simulink model "MBNLC_cascade_rov"  (Simulink 6.0)
settings: Solver=ode45  StartTime=0.0  StopTime=650  RelTol=1e-3
undefined symbols (not defined in the file): B, DQ, DQL, I, m, M, Ma, MaL, MaU, rg, sigbuilder_block, T, W, xb, xg, Xudot, yb, yg, Yvdot, zb, zg, Zwdot
libraries: simulink_extras x12, simulink x8
(part 3 of 3)

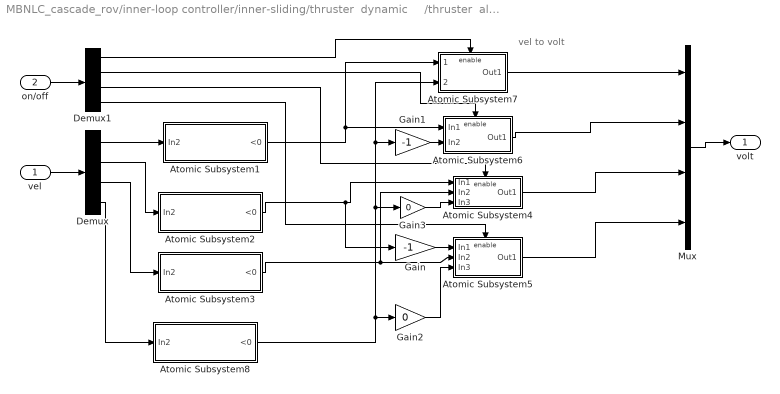
== system MBNLC_cascade_rov/inner-loop controller/inner-sliding/thruster  dynamic     /thruster  alloc. /thruster  allocation control1/thruster allocation  ==
  note: vel to volt
  vel : Inport  Port=1  LatchInput=off
  on/off : Inport  Port=2  LatchInput=off
  Atomic Subsystem1 : Subsystem  TreatAsAtomicUnit=on
      mask Display: disp('check x >0, send \n signal to thrusters ')
  Atomic Subsystem2 : Subsystem  TreatAsAtomicUnit=on
      mask Display: disp('check y >0, send \n signal to thrusters ')
  Atomic Subsystem3 : Subsystem  TreatAsAtomicUnit=on
      mask Display: disp('check z >0, send \n signal to thrusters ')
  Atomic Subsystem4 : Subsystem  TreatAsAtomicUnit=on
      mask Display: disp('activate T3')
  Atomic Subsystem5 : Subsystem  TreatAsAtomicUnit=on
      mask Display: disp('activate T4')
  Atomic Subsystem6 : Subsystem  TreatAsAtomicUnit=on
      mask Display: disp('activate T2')
  Atomic Subsystem7 : Subsystem  TreatAsAtomicUnit=on
      mask Display: disp('activate T1')
  Atomic Subsystem8 : Subsystem  TreatAsAtomicUnit=on
      mask Display: disp('check yaw >0, send \n signal to thrusters ')
  Demux : Demux
  Demux1 : Demux
  Gain : Gain  Gain=-1
  Gain1 : Gain  Gain=-1
  Gain2 : Gain  Gain=0
  Gain3 : Gain  Gain=0
  Mux : Mux
  volt : Outport
  wires:
  Demux/1 -> Atomic Subsystem1/1(In2)
  Demux/2 -> Atomic Subsystem2/1(In2)
  Demux/3 -> Atomic Subsystem3/1(In2)
  Atomic Subsystem7/1(Out1) -> Mux/1
  vel/1 -> Demux/1
  Demux/4 -> Atomic Subsystem8/1(In2)
  on/off/1 -> Demux1/1
  Mux/1 -> volt/1
  Atomic Subsystem6/1(Out1) -> Mux/2
  Atomic Subsystem4/1(Out1) -> Mux/3
  Atomic Subsystem5/1(Out1) -> Mux/4
  Atomic Subsystem1/1(<0) -> Atomic Subsystem7/1(1), Atomic Subsystem6/1(In1)
  Atomic Subsystem2/1(<0) -> Atomic Subsystem4/1(In1), Gain/1
  Atomic Subsystem3/1(<0) -> Atomic Subsystem4/2(In2), Atomic Subsystem5/2(In2)
  Gain/1 -> Atomic Subsystem5/1(In1)
  Atomic Subsystem8/1(<0) -> Atomic Subsystem7/2(2), Gain1/1, Gain3/1, Gain2/1
  Gain1/1 -> Atomic Subsystem6/2(In2)
  Gain2/1 -> Atomic Subsystem5/3(In3)
  Demux1/1 -> Atomic Subsystem7/Enable
  Demux1/2 -> Atomic Subsystem6/Enable
  Demux1/3 -> Atomic Subsystem4/Enable
  Demux1/4 -> Atomic Subsystem5/Enable
  Gain3/1 -> Atomic Subsystem4/3(In3)

== system MBNLC_cascade_rov/inner-loop controller/inner -PI-decouple /thruster  dynamic     /thruster  alloc. /thruster  allocation control1/thruster allocation /Atomic Subsystem1 ==
  In2 : Inport  Port=1  LatchInput=off
  Abs : Abs
  Product1 : Product  OutDataTypeMode=double  SaturateOnIntegerOverflow=on  RndMeth=Zero
  Product5 : Product  OutDataTypeMode=double  SaturateOnIntegerOverflow=on  RndMeth=Zero
  Sign1 : Signum
  Switch1 : Switch  Threshold=1  SaturateOnIntegerOverflow=on  InputSameDT=on
  <0 : Outport
  wires:
  Sign1/1 -> Product1/2, Product5/1, Switch1/2
  Product1/1 -> Switch1/1
  Product5/1 -> Switch1/3
  Switch1/1 -> <0/1
  In2/1 -> Sign1/1, Product1/1, Abs/1
  Abs/1 -> Product5/2

== system MBNLC_cascade_rov/inner-loop controller/inner -PI-decouple /thruster  dynamic     /thruster  alloc. /thruster  allocation control1/thruster allocation /Atomic Subsystem2 ==
  In2 : Inport  Port=1  LatchInput=off
  Abs : Abs
  Product1 : Product  OutDataTypeMode=double  SaturateOnIntegerOverflow=on  RndMeth=Zero
  Product5 : Product  OutDataTypeMode=double  SaturateOnIntegerOverflow=on  RndMeth=Zero
  Sign1 : Signum
  Switch1 : Switch  Threshold=1  SaturateOnIntegerOverflow=on  InputSameDT=on
  <0 : Outport
  wires:
  In2/1 -> Sign1/1, Product1/1, Abs/1
  Sign1/1 -> Switch1/2, Product1/2, Product5/1
  Product1/1 -> Switch1/1
  Product5/1 -> Switch1/3
  Switch1/1 -> <0/1
  Abs/1 -> Product5/2

== system MBNLC_cascade_rov/inner-loop controller/inner -PI-decouple /thruster  dynamic     /thruster  alloc. /thruster  allocation control1/thruster allocation /Atomic Subsystem3 ==
  In2 : Inport  Port=1  LatchInput=off
  Abs : Abs
  Product1 : Product  OutDataTypeMode=double  SaturateOnIntegerOverflow=on  RndMeth=Zero
  Product5 : Product  OutDataTypeMode=double  SaturateOnIntegerOverflow=on  RndMeth=Zero
  Sign1 : Signum
  Switch1 : Switch  Threshold=1  SaturateOnIntegerOverflow=on  InputSameDT=on
  <0 : Outport
  wires:
  Sign1/1 -> Switch1/2, Product1/2, Product5/1
  Product1/1 -> Switch1/1
  Product5/1 -> Switch1/3
  Switch1/1 -> <0/1
  In2/1 -> Sign1/1, Product1/1, Abs/1
  Abs/1 -> Product5/2

== system MBNLC_cascade_rov/inner-loop controller/inner -PI-decouple /thruster  dynamic     /thruster  alloc. /thruster  allocation control1/thruster allocation /Atomic Subsystem4 ==
  In1 : Inport  Port=1  LatchInput=off
  In2 : Inport  Port=2  LatchInput=off
  In3 : Inport  Port=3  LatchInput=off
  Enable : EnablePort
  Subtract : Sum  Inputs=+++  OutScaling=2^-10
  Out1 : Outport
  wires:
  In1/1 -> Subtract/1
  In2/1 -> Subtract/2
  In3/1 -> Subtract/3
  Subtract/1 -> Out1/1

== system MBNLC_cascade_rov/inner-loop controller/inner -PI-decouple /thruster  dynamic     /thruster  alloc. /thruster  allocation control1/thruster allocation /Atomic Subsystem5 ==
  In1 : Inport  Port=1  LatchInput=off
  In2 : Inport  Port=2  LatchInput=off
  In3 : Inport  Port=3  LatchInput=off
  Enable : EnablePort
  Subtract : Sum  Inputs=+++  OutScaling=2^-10
  Out1 : Outport
  wires:
  In1/1 -> Subtract/1
  In2/1 -> Subtract/2
  In3/1 -> Subtract/3
  Subtract/1 -> Out1/1

== system MBNLC_cascade_rov/inner-loop controller/inner -PI-decouple /thruster  dynamic     /thruster  alloc. /thruster  allocation control1/thruster allocation /Atomic Subsystem6 ==
  In1 : Inport  Port=1  LatchInput=off
  In2 : Inport  Port=2  LatchInput=off
  Enable : EnablePort
  Subtract : Sum  OutScaling=2^-10
  Out1 : Outport
  wires:
  In1/1 -> Subtract/1
  In2/1 -> Subtract/2
  Subtract/1 -> Out1/1

== system MBNLC_cascade_rov/inner-loop controller/inner -PI-decouple /thruster  dynamic     /thruster  alloc. /thruster  allocation control1/thruster allocation /Atomic Subsystem7 ==
  1 : Inport  Port=1  LatchInput=off
  2 : Inport  Port=2  LatchInput=off
  Enable : EnablePort
  Subtract : Sum  OutScaling=2^-10
  Out1 : Outport
  wires:
  1/1 -> Subtract/1
  2/1 -> Subtract/2
  Subtract/1 -> Out1/1

== system MBNLC_cascade_rov/inner-loop controller/inner -PI-decouple /thruster  dynamic     /thruster  alloc. /thruster  allocation control1/thruster allocation /Atomic Subsystem8 ==
  In2 : Inport  Port=1  LatchInput=off
  Abs : Abs
  Product1 : Product  OutDataTypeMode=double  SaturateOnIntegerOverflow=on  RndMeth=Zero
  Product5 : Product  OutDataTypeMode=double  SaturateOnIntegerOverflow=on  RndMeth=Zero
  Sign1 : Signum
  Switch1 : Switch  Threshold=1  SaturateOnIntegerOverflow=on  InputSameDT=on
  <0 : Outport
  wires:
  In2/1 -> Sign1/1, Product1/1, Abs/1
  Sign1/1 -> Switch1/2, Product1/2, Product5/1
  Product1/1 -> Switch1/1
  Product5/1 -> Switch1/3
  Switch1/1 -> <0/1
  Abs/1 -> Product5/2

== system MBNLC_cascade_rov/inner-loop controller/inner -backstepping/thruster  dynamic     /thruster  alloc. /thruster  allocation control1/thruster allocation /Atomic Subsystem1 ==
  In2 : Inport  Port=1  LatchInput=off
  Abs : Abs
  Product1 : Product  OutDataTypeMode=double  SaturateOnIntegerOverflow=on  RndMeth=Zero
  Product5 : Product  OutDataTypeMode=double  SaturateOnIntegerOverflow=on  RndMeth=Zero
  Sign1 : Signum
  Switch1 : Switch  Threshold=1  SaturateOnIntegerOverflow=on  InputSameDT=on
  <0 : Outport
  wires:
  Sign1/1 -> Product1/2, Product5/1, Switch1/2
  Product1/1 -> Switch1/1
  Product5/1 -> Switch1/3
  Switch1/1 -> <0/1
  In2/1 -> Sign1/1, Product1/1, Abs/1
  Abs/1 -> Product5/2

== system MBNLC_cascade_rov/inner-loop controller/inner -backstepping/thruster  dynamic     /thruster  alloc. /thruster  allocation control1/thruster allocation /Atomic Subsystem2 ==
  In2 : Inport  Port=1  LatchInput=off
  Abs : Abs
  Product1 : Product  OutDataTypeMode=double  SaturateOnIntegerOverflow=on  RndMeth=Zero
  Product5 : Product  OutDataTypeMode=double  SaturateOnIntegerOverflow=on  RndMeth=Zero
  Sign1 : Signum
  Switch1 : Switch  Threshold=1  SaturateOnIntegerOverflow=on  InputSameDT=on
  <0 : Outport
  wires:
  In2/1 -> Sign1/1, Product1/1, Abs/1
  Sign1/1 -> Switch1/2, Product1/2, Product5/1
  Product1/1 -> Switch1/1
  Product5/1 -> Switch1/3
  Switch1/1 -> <0/1
  Abs/1 -> Product5/2

== system MBNLC_cascade_rov/inner-loop controller/inner -backstepping/thruster  dynamic     /thruster  alloc. /thruster  allocation control1/thruster allocation /Atomic Subsystem3 ==
  In2 : Inport  Port=1  LatchInput=off
  Abs : Abs
  Product1 : Product  OutDataTypeMode=double  SaturateOnIntegerOverflow=on  RndMeth=Zero
  Product5 : Product  OutDataTypeMode=double  SaturateOnIntegerOverflow=on  RndMeth=Zero
  Sign1 : Signum
  Switch1 : Switch  Threshold=1  SaturateOnIntegerOverflow=on  InputSameDT=on
  <0 : Outport
  wires:
  Sign1/1 -> Switch1/2, Product1/2, Product5/1
  Product1/1 -> Switch1/1
  Product5/1 -> Switch1/3
  Switch1/1 -> <0/1
  In2/1 -> Sign1/1, Product1/1, Abs/1
  Abs/1 -> Product5/2

== system MBNLC_cascade_rov/inner-loop controller/inner -backstepping/thruster  dynamic     /thruster  alloc. /thruster  allocation control1/thruster allocation /Atomic Subsystem4 ==
  In1 : Inport  Port=1  LatchInput=off
  In2 : Inport  Port=2  LatchInput=off
  In3 : Inport  Port=3  LatchInput=off
  Enable : EnablePort
  Subtract : Sum  Inputs=+++  OutScaling=2^-10
  Out1 : Outport
  wires:
  In1/1 -> Subtract/1
  In2/1 -> Subtract/2
  In3/1 -> Subtract/3
  Subtract/1 -> Out1/1

== system MBNLC_cascade_rov/inner-loop controller/inner -backstepping/thruster  dynamic     /thruster  alloc. /thruster  allocation control1/thruster allocation /Atomic Subsystem5 ==
  In1 : Inport  Port=1  LatchInput=off
  In2 : Inport  Port=2  LatchInput=off
  In3 : Inport  Port=3  LatchInput=off
  Enable : EnablePort
  Subtract : Sum  Inputs=+++  OutScaling=2^-10
  Out1 : Outport
  wires:
  In1/1 -> Subtract/1
  In2/1 -> Subtract/2
  In3/1 -> Subtract/3
  Subtract/1 -> Out1/1

== system MBNLC_cascade_rov/inner-loop controller/inner -backstepping/thruster  dynamic     /thruster  alloc. /thruster  allocation control1/thruster allocation /Atomic Subsystem6 ==
  In1 : Inport  Port=1  LatchInput=off
  In2 : Inport  Port=2  LatchInput=off
  Enable : EnablePort
  Subtract : Sum  OutScaling=2^-10
  Out1 : Outport
  wires:
  In1/1 -> Subtract/1
  In2/1 -> Subtract/2
  Subtract/1 -> Out1/1

== system MBNLC_cascade_rov/inner-loop controller/inner -backstepping/thruster  dynamic     /thruster  alloc. /thruster  allocation control1/thruster allocation /Atomic Subsystem7 ==
  1 : Inport  Port=1  LatchInput=off
  2 : Inport  Port=2  LatchInput=off
  Enable : EnablePort
  Subtract : Sum  OutScaling=2^-10
  Out1 : Outport
  wires:
  1/1 -> Subtract/1
  2/1 -> Subtract/2
  Subtract/1 -> Out1/1

== system MBNLC_cascade_rov/inner-loop controller/inner -backstepping/thruster  dynamic     /thruster  alloc. /thruster  allocation control1/thruster allocation /Atomic Subsystem8 ==
  In2 : Inport  Port=1  LatchInput=off
  Abs : Abs
  Product1 : Product  OutDataTypeMode=double  SaturateOnIntegerOverflow=on  RndMeth=Zero
  Product5 : Product  OutDataTypeMode=double  SaturateOnIntegerOverflow=on  RndMeth=Zero
  Sign1 : Signum
  Switch1 : Switch  Threshold=1  SaturateOnIntegerOverflow=on  InputSameDT=on
  <0 : Outport
  wires:
  In2/1 -> Sign1/1, Product1/1, Abs/1
  Sign1/1 -> Switch1/2, Product1/2, Product5/1
  Product1/1 -> Switch1/1
  Product5/1 -> Switch1/3
  Switch1/1 -> <0/1
  Abs/1 -> Product5/2

== system MBNLC_cascade_rov/inner-loop controller/inner-P/thruster  dynamic     /thruster  alloc. /thruster  allocation control1/thruster allocation /Atomic Subsystem1 ==
  In2 : Inport  Port=1  LatchInput=off
  Abs : Abs
  Product1 : Product  OutDataTypeMode=double  SaturateOnIntegerOverflow=on  RndMeth=Zero
  Product5 : Product  OutDataTypeMode=double  SaturateOnIntegerOverflow=on  RndMeth=Zero
  Sign1 : Signum
  Switch1 : Switch  Threshold=1  SaturateOnIntegerOverflow=on  InputSameDT=on
  <0 : Outport
  wires:
  Sign1/1 -> Product1/2, Product5/1, Switch1/2
  Product1/1 -> Switch1/1
  Product5/1 -> Switch1/3
  Switch1/1 -> <0/1
  In2/1 -> Sign1/1, Product1/1, Abs/1
  Abs/1 -> Product5/2

== system MBNLC_cascade_rov/inner-loop controller/inner-P/thruster  dynamic     /thruster  alloc. /thruster  allocation control1/thruster allocation /Atomic Subsystem2 ==
  In2 : Inport  Port=1  LatchInput=off
  Abs : Abs
  Product1 : Product  OutDataTypeMode=double  SaturateOnIntegerOverflow=on  RndMeth=Zero
  Product5 : Product  OutDataTypeMode=double  SaturateOnIntegerOverflow=on  RndMeth=Zero
  Sign1 : Signum
  Switch1 : Switch  Threshold=1  SaturateOnIntegerOverflow=on  InputSameDT=on
  <0 : Outport
  wires:
  In2/1 -> Sign1/1, Product1/1, Abs/1
  Sign1/1 -> Switch1/2, Product1/2, Product5/1
  Product1/1 -> Switch1/1
  Product5/1 -> Switch1/3
  Switch1/1 -> <0/1
  Abs/1 -> Product5/2

== system MBNLC_cascade_rov/inner-loop controller/inner-P/thruster  dynamic     /thruster  alloc. /thruster  allocation control1/thruster allocation /Atomic Subsystem3 ==
  In2 : Inport  Port=1  LatchInput=off
  Abs : Abs
  Product1 : Product  OutDataTypeMode=double  SaturateOnIntegerOverflow=on  RndMeth=Zero
  Product5 : Product  OutDataTypeMode=double  SaturateOnIntegerOverflow=on  RndMeth=Zero
  Sign1 : Signum
  Switch1 : Switch  Threshold=1  SaturateOnIntegerOverflow=on  InputSameDT=on
  <0 : Outport
  wires:
  Sign1/1 -> Switch1/2, Product1/2, Product5/1
  Product1/1 -> Switch1/1
  Product5/1 -> Switch1/3
  Switch1/1 -> <0/1
  In2/1 -> Sign1/1, Product1/1, Abs/1
  Abs/1 -> Product5/2

== system MBNLC_cascade_rov/inner-loop controller/inner-P/thruster  dynamic     /thruster  alloc. /thruster  allocation control1/thruster allocation /Atomic Subsystem4 ==
  In1 : Inport  Port=1  LatchInput=off
  In2 : Inport  Port=2  LatchInput=off
  In3 : Inport  Port=3  LatchInput=off
  Enable : EnablePort
  Subtract : Sum  Inputs=+++  OutScaling=2^-10
  Out1 : Outport
  wires:
  In1/1 -> Subtract/1
  In2/1 -> Subtract/2
  In3/1 -> Subtract/3
  Subtract/1 -> Out1/1

== system MBNLC_cascade_rov/inner-loop controller/inner-P/thruster  dynamic     /thruster  alloc. /thruster  allocation control1/thruster allocation /Atomic Subsystem5 ==
  In1 : Inport  Port=1  LatchInput=off
  In2 : Inport  Port=2  LatchInput=off
  In3 : Inport  Port=3  LatchInput=off
  Enable : EnablePort
  Subtract : Sum  Inputs=+++  OutScaling=2^-10
  Out1 : Outport
  wires:
  In1/1 -> Subtract/1
  In2/1 -> Subtract/2
  In3/1 -> Subtract/3
  Subtract/1 -> Out1/1

== system MBNLC_cascade_rov/inner-loop controller/inner-P/thruster  dynamic     /thruster  alloc. /thruster  allocation control1/thruster allocation /Atomic Subsystem6 ==
  In1 : Inport  Port=1  LatchInput=off
  In2 : Inport  Port=2  LatchInput=off
  Enable : EnablePort
  Subtract : Sum  OutScaling=2^-10
  Out1 : Outport
  wires:
  In1/1 -> Subtract/1
  In2/1 -> Subtract/2
  Subtract/1 -> Out1/1

== system MBNLC_cascade_rov/inner-loop controller/inner-P/thruster  dynamic     /thruster  alloc. /thruster  allocation control1/thruster allocation /Atomic Subsystem7 ==
  1 : Inport  Port=1  LatchInput=off
  2 : Inport  Port=2  LatchInput=off
  Enable : EnablePort
  Subtract : Sum  OutScaling=2^-10
  Out1 : Outport
  wires:
  1/1 -> Subtract/1
  2/1 -> Subtract/2
  Subtract/1 -> Out1/1

== system MBNLC_cascade_rov/inner-loop controller/inner-P/thruster  dynamic     /thruster  alloc. /thruster  allocation control1/thruster allocation /Atomic Subsystem8 ==
  In2 : Inport  Port=1  LatchInput=off
  Abs : Abs
  Product1 : Product  OutDataTypeMode=double  SaturateOnIntegerOverflow=on  RndMeth=Zero
  Product5 : Product  OutDataTypeMode=double  SaturateOnIntegerOverflow=on  RndMeth=Zero
  Sign1 : Signum
  Switch1 : Switch  Threshold=1  SaturateOnIntegerOverflow=on  InputSameDT=on
  <0 : Outport
  wires:
  In2/1 -> Sign1/1, Product1/1, Abs/1
  Sign1/1 -> Switch1/2, Product1/2, Product5/1
  Product1/1 -> Switch1/1
  Product5/1 -> Switch1/3
  Switch1/1 -> <0/1
  Abs/1 -> Product5/2

== system MBNLC_cascade_rov/inner-loop controller/inner-sliding/thruster  dynamic     /thruster  alloc. /thruster  allocation control1/thruster allocation /Atomic Subsystem1 ==
  In2 : Inport  Port=1  LatchInput=off
  Abs : Abs
  Product1 : Product  OutDataTypeMode=double  SaturateOnIntegerOverflow=on  RndMeth=Zero
  Product5 : Product  OutDataTypeMode=double  SaturateOnIntegerOverflow=on  RndMeth=Zero
  Sign1 : Signum
  Switch1 : Switch  Threshold=1  SaturateOnIntegerOverflow=on  InputSameDT=on
  <0 : Outport
  wires:
  Sign1/1 -> Product1/2, Product5/1, Switch1/2
  Product1/1 -> Switch1/1
  Product5/1 -> Switch1/3
  Switch1/1 -> <0/1
  In2/1 -> Sign1/1, Product1/1, Abs/1
  Abs/1 -> Product5/2

== system MBNLC_cascade_rov/inner-loop controller/inner-sliding/thruster  dynamic     /thruster  alloc. /thruster  allocation control1/thruster allocation /Atomic Subsystem2 ==
  In2 : Inport  Port=1  LatchInput=off
  Abs : Abs
  Product1 : Product  OutDataTypeMode=double  SaturateOnIntegerOverflow=on  RndMeth=Zero
  Product5 : Product  OutDataTypeMode=double  SaturateOnIntegerOverflow=on  RndMeth=Zero
  Sign1 : Signum
  Switch1 : Switch  Threshold=1  SaturateOnIntegerOverflow=on  InputSameDT=on
  <0 : Outport
  wires:
  In2/1 -> Sign1/1, Product1/1, Abs/1
  Sign1/1 -> Switch1/2, Product1/2, Product5/1
  Product1/1 -> Switch1/1
  Product5/1 -> Switch1/3
  Switch1/1 -> <0/1
  Abs/1 -> Product5/2

== system MBNLC_cascade_rov/inner-loop controller/inner-sliding/thruster  dynamic     /thruster  alloc. /thruster  allocation control1/thruster allocation /Atomic Subsystem3 ==
  In2 : Inport  Port=1  LatchInput=off
  Abs : Abs
  Product1 : Product  OutDataTypeMode=double  SaturateOnIntegerOverflow=on  RndMeth=Zero
  Product5 : Product  OutDataTypeMode=double  SaturateOnIntegerOverflow=on  RndMeth=Zero
  Sign1 : Signum
  Switch1 : Switch  Threshold=1  SaturateOnIntegerOverflow=on  InputSameDT=on
  <0 : Outport
  wires:
  Sign1/1 -> Switch1/2, Product1/2, Product5/1
  Product1/1 -> Switch1/1
  Product5/1 -> Switch1/3
  Switch1/1 -> <0/1
  In2/1 -> Sign1/1, Product1/1, Abs/1
  Abs/1 -> Product5/2

== system MBNLC_cascade_rov/inner-loop controller/inner-sliding/thruster  dynamic     /thruster  alloc. /thruster  allocation control1/thruster allocation /Atomic Subsystem4 ==
  In1 : Inport  Port=1  LatchInput=off
  In2 : Inport  Port=2  LatchInput=off
  In3 : Inport  Port=3  LatchInput=off
  Enable : EnablePort
  Subtract : Sum  Inputs=+++  OutScaling=2^-10
  Out1 : Outport
  wires:
  In1/1 -> Subtract/1
  In2/1 -> Subtract/2
  In3/1 -> Subtract/3
  Subtract/1 -> Out1/1

== system MBNLC_cascade_rov/inner-loop controller/inner-sliding/thruster  dynamic     /thruster  alloc. /thruster  allocation control1/thruster allocation /Atomic Subsystem5 ==
  In1 : Inport  Port=1  LatchInput=off
  In2 : Inport  Port=2  LatchInput=off
  In3 : Inport  Port=3  LatchInput=off
  Enable : EnablePort
  Subtract : Sum  Inputs=+++  OutScaling=2^-10
  Out1 : Outport
  wires:
  In1/1 -> Subtract/1
  In2/1 -> Subtract/2
  In3/1 -> Subtract/3
  Subtract/1 -> Out1/1

== system MBNLC_cascade_rov/inner-loop controller/inner-sliding/thruster  dynamic     /thruster  alloc. /thruster  allocation control1/thruster allocation /Atomic Subsystem6 ==
  In1 : Inport  Port=1  LatchInput=off
  In2 : Inport  Port=2  LatchInput=off
  Enable : EnablePort
  Subtract : Sum  OutScaling=2^-10
  Out1 : Outport
  wires:
  In1/1 -> Subtract/1
  In2/1 -> Subtract/2
  Subtract/1 -> Out1/1

== system MBNLC_cascade_rov/inner-loop controller/inner-sliding/thruster  dynamic     /thruster  alloc. /thruster  allocation control1/thruster allocation /Atomic Subsystem7 ==
  1 : Inport  Port=1  LatchInput=off
  2 : Inport  Port=2  LatchInput=off
  Enable : EnablePort
  Subtract : Sum  OutScaling=2^-10
  Out1 : Outport
  wires:
  1/1 -> Subtract/1
  2/1 -> Subtract/2
  Subtract/1 -> Out1/1

== system MBNLC_cascade_rov/inner-loop controller/inner-sliding/thruster  dynamic     /thruster  alloc. /thruster  allocation control1/thruster allocation /Atomic Subsystem8 ==
  In2 : Inport  Port=1  LatchInput=off
  Abs : Abs
  Product1 : Product  OutDataTypeMode=double  SaturateOnIntegerOverflow=on  RndMeth=Zero
  Product5 : Product  OutDataTypeMode=double  SaturateOnIntegerOverflow=on  RndMeth=Zero
  Sign1 : Signum
  Switch1 : Switch  Threshold=1  SaturateOnIntegerOverflow=on  InputSameDT=on
  <0 : Outport
  wires:
  In2/1 -> Sign1/1, Product1/1, Abs/1
  Sign1/1 -> Switch1/2, Product1/2, Product5/1
  Product1/1 -> Switch1/1
  Product5/1 -> Switch1/3
  Switch1/1 -> <0/1
  Abs/1 -> Product5/2
